simulink model "model_wielomianowy_dynamika"  (R2014b)
settings: Solver=ode23  StartTime=0.0  StopTime=10.0  RelTol=1e-3
values from neighbouring files (symbols this model uses):
  b0 = (x1T-x10)/T    (= 0.1)    [wielomianowy.m]
  c = [b0*T^3/6, -T^2/2; -b0*T^2/2, T]*[xT(2)-xz(2); xT(3)-xz(3)-b0*xz(2)*T]*-12/(b0*T^4)    [wielomianowy.m]
  K = 100    [dynamika.m]    (also in monocykl.m)
  M11 = Mc+2*Mk*L*L    (= 107.9)    [dynamika.m]    (also in monocykl.m; wielomianowy.m)
  M22 = Ip/(L*L)    (= 83.5895833333)    [dynamika.m]    (also in monocykl.m; wielomianowy.m)
  teta0 = 0    [dynamika.m]    (also in kinematyka.m; monocykl.m = 3; wielomianowy.m)
  v0 = 1    [monocykl.m]    (also in wielomianowy.m = 0)
  w0 = 10    [monocykl.m]    (also in wielomianowy.m = 0)
  x0 = 0    [dynamika.m]    (also in kinematyka.m; monocykl.m = 4; wielomianowy.m = 1)
  y0 = 0    [dynamika.m]    (also in kinematyka.m; monocykl.m = 2; wielomianowy.m = 2)
settings Model: Creator=Dawid Perdek  LastModifiedBy=Dawid Perdek

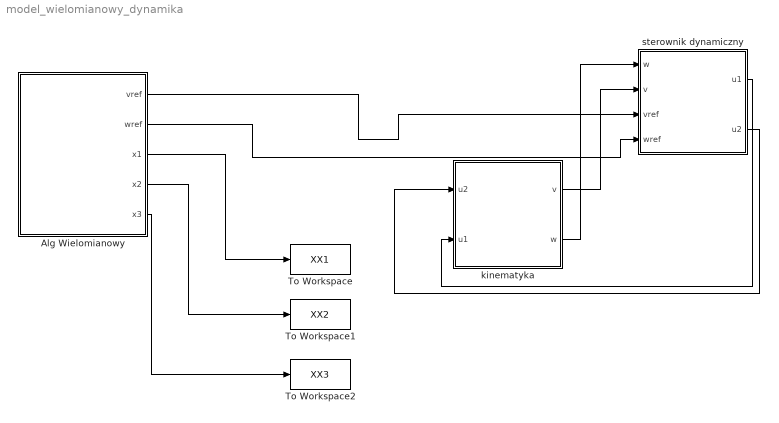
== system model_wielomianowy_dynamika ==
  Alg Wielomianowy : Subsystem
  To Workspace : ToWorkspace  VariableName=XX1  SampleTime=-1
  To Workspace1 : ToWorkspace  VariableName=XX2  SampleTime=-1
  To Workspace2 : ToWorkspace  VariableName=XX3  SampleTime=-1
  kinematyka : Subsystem
  sterownik dynamiczny : Subsystem
  wires:
  Alg Wielomianowy/2(wref) -> sterownik dynamiczny/4(wref)
  Alg Wielomianowy/1(vref) -> sterownik dynamiczny/3(vref)
  kinematyka/1(v) -> sterownik dynamiczny/2(v)
  kinematyka/2(w) -> sterownik dynamiczny/1(w)
  Alg Wielomianowy/3(x1) -> To Workspace/1
  Alg Wielomianowy/5(x3) -> To Workspace2/1
  Alg Wielomianowy/4(x2) -> To Workspace1/1
  sterownik dynamiczny/2(u2) -> kinematyka/1(u2)
  sterownik dynamiczny/1(u1) -> kinematyka/2(u1)

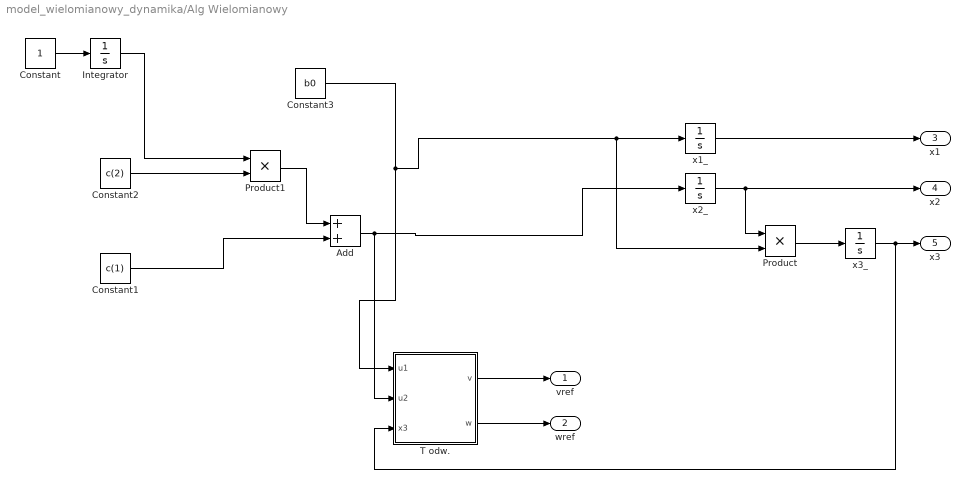
== system model_wielomianowy_dynamika/Alg Wielomianowy ==
  Add : Sum
  Constant : Constant
  Constant1 : Constant  Value=c(1)
  Constant2 : Constant  Value=c(2)
  Constant3 : Constant  Value=b0
  Integrator : Integrator
  Product : Product
  Product1 : Product
  T odw. : Subsystem
  x1_ : Integrator
  x2_ : Integrator  InitialCondition=-1
  x3_ : Integrator  InitialCondition=2
  vref : Outport
  wref : Outport  Port=2
  x1 : Outport  Port=3
  x2 : Outport  Port=4
  x3 : Outport  Port=5
  wires:
  Constant/1 -> Integrator/1
  Integrator/1 -> Product1/1
  Constant2/1 -> Product1/2
  Product1/1 -> Add/1
  Constant1/1 -> Add/2
  Add/1 -> T odw./2(u2), x2_/1
  Constant3/1 -> T odw./1(u1), Product/2, x1_/1
  T odw./2(w) -> wref/1
  T odw./1(v) -> vref/1
  x2_/1 -> x2/1, Product/1
  x1_/1 -> x1/1
  x3_/1 -> T odw./3(x3), x3/1
  Product/1 -> x3_/1

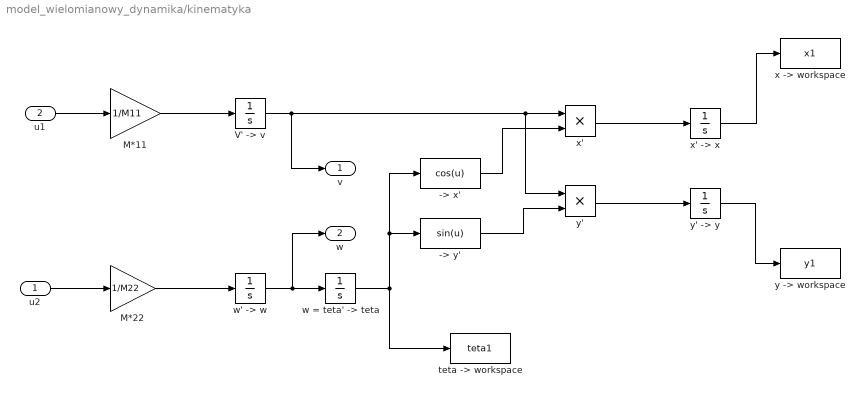
== system model_wielomianowy_dynamika/kinematyka ==
  u2 : Inport
  u1 : Inport  Port=2
  -> x' : Fcn  Expr=cos(u)
  -> y' : Fcn  Expr=sin(u)
  M*11 : Gain  Gain=1/M11
  M*22 : Gain  Gain=1/M22
  "V' -> v" : Integrator  InitialCondition=v0
  "teta -> workspace" : ToWorkspace  VariableName=teta1  SampleTime=-1
  "w = teta' -> teta" : Integrator  InitialCondition=teta0
  "w' -> w" : Integrator  InitialCondition=w0
  "x -> workspace" : ToWorkspace  VariableName=x1  SampleTime=-1
  x' : Product
  "x' -> x" : Integrator  InitialCondition=x0
  "y -> workspace" : ToWorkspace  VariableName=y1  SampleTime=-1
  y' : Product
  "y' -> y" : Integrator  InitialCondition=y0
  v : Outport
  w : Outport  Port=2
  wires:
  u2/1 -> M*22/1
  u1/1 -> M*11/1
  -> x'/1 -> x'/2
  -> y'/1 -> y'/2
  x'/1 -> "x' -> x"/1
  y'/1 -> "y' -> y"/1
  "x' -> x"/1 -> "x -> workspace"/1
  "y' -> y"/1 -> "y -> workspace"/1
  "w = teta' -> teta"/1 -> "teta -> workspace"/1, -> x'/1, -> y'/1
  M*11/1 -> "V' -> v"/1
  "V' -> v"/1 -> v/1, y'/1, x'/1
  M*22/1 -> "w' -> w"/1
  "w' -> w"/1 -> w/1, "w = teta' -> teta"/1

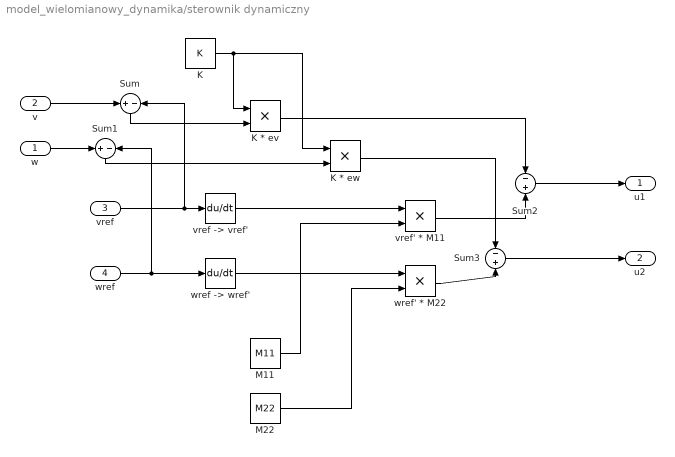
== system model_wielomianowy_dynamika/sterownik dynamiczny ==
  w : Inport
  v : Inport  Port=2
  vref : Inport  Port=3
  wref : Inport  Port=4
  K : Constant  Value=K
  K * ev : Product
  K * ew : Product
  M11 : Constant  Value=M11
  M22 : Constant  Value=M22
  Sum : Sum  Inputs=+-
  Sum1 : Sum  Inputs=+-
  Sum2 : Sum  Inputs=-+
  Sum3 : Sum  Inputs=-+
  "vref -> vref'" : Derivative
  vref' * M11 : Product
  "wref -> wref'" : Derivative
  wref' * M22 : Product
  u1 : Outport
  u2 : Outport  Port=2
  wires:
  vref/1 -> Sum/2, "vref -> vref'"/1
  wref/1 -> Sum1/2, "wref -> wref'"/1
  "vref -> vref'"/1 -> vref' * M11/1
  M11/1 -> vref' * M11/2
  "wref -> wref'"/1 -> wref' * M22/1
  M22/1 -> wref' * M22/2
  v/1 -> Sum/1
  w/1 -> Sum1/1
  Sum/1 -> K * ev/2
  Sum1/1 -> K * ew/2
  K/1 -> K * ew/1, K * ev/1
  vref' * M11/1 -> Sum2/2
  K * ev/1 -> Sum2/1
  wref' * M22/1 -> Sum3/2
  K * ew/1 -> Sum3/1
  Sum2/1 -> u1/1
  Sum3/1 -> u2/1

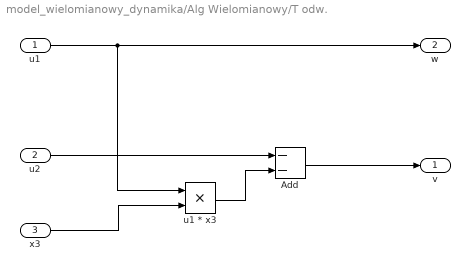
== system model_wielomianowy_dynamika/Alg Wielomianowy/T odw. ==
  u1 : Inport
  u2 : Inport  Port=2
  x3 : Inport  Port=3
  Add : Sum  Inputs=--
  u1 * x3 : Product
  v : Outport
  w : Outport  Port=2
  wires:
  u1/1 -> w/1, u1 * x3/1
  x3/1 -> u1 * x3/2
  u1 * x3/1 -> Add/2
  u2/1 -> Add/1
  Add/1 -> v/1
